simulink model "persistent_test"  (R2014a)
settings: Solver=ode3  StartTime=0.0  StopTime=10.0  FixedStep=1  RelTol=1e-3
settings Model: Creator=mariutho  LastModifiedBy=mariutho

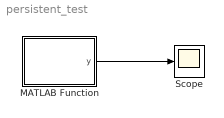
== system persistent_test ==
  MATLAB Function : MATLAB Function  TreatAsAtomicUnit=on
  Scope : Scope
  wires:
  MATLAB Function/1(y) -> Scope/1

== matlab function persistent_test/MATLAB Function ==
  data: y output
function y = fcn()
	persistent x
	if isempty(x)
		x = 0;
	else
		x = x+1;
	end
	

y = x;
